simulink model "inverted_pendulum"  (R2021a)
settings: Solver=ode15s  StartTime=0.0  StopTime=35  FixedStep=0.1  RelTol=1e-3  EnableMultiTasking=on
settings Model: Creator=glembrez  LastModifiedBy=gabin
settings SolverCC: AlgebraicLoopSolver=TrustRegion  AutoInsertRateTranBlk=on
settings DataIOCC: LimitDataPoints=on
settings OptimizationCC: LifeSpan=inf
settings DebuggingCC: AllowSymbolicDim=off  SFUnexpectedBacktrackingDiag=warning  SFNoUnconditionalDefaultTransitionDiag=warning  SFExecutionAtInitializationDiag=none  ArithmeticOperatorsInVariantConditions=warning
settings SFSimCC: SimUseLocalCustomCode=off  CustomCodeUndefinedFunction=UseInterfaceOnly
settings RTWCC: RTWUseLocalCustomCode=off
settings CodeAppCC: StateflowObjectComments=on
settings GRTTargetCC: TargetLangStandard=C89/C90 (ANSI)
settings ConfigComp: CovMetricSettings=dw  CovSaveCumulativeToWorkspaceVar=on  CovSaveSingleToWorkspaceVar=on  CovExternalEMLEnable=off  CovSFcnEnable=off

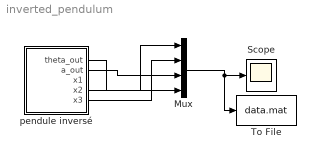
== system inverted_pendulum ==
  Mux : Mux
  Scope : Scope
  To File : ToFile  Filename=data.mat  MatrixName=X  SaveFormat=Timeseries
  pendule inversé : Stateflow chart  TreatAsAtomicUnit=on
  wires:
  Mux/1 -> Scope/1, To File/1
  pendule inversé/1(theta_out) -> Mux/4
  pendule inversé/2(a_out) -> Mux/3
  pendule inversé/4(x2) -> Mux/1
  pendule inversé/5(x3) -> Mux/2

== stateflow chart inverted_pendulum/pendule inversé ==
  settings: updateMethod=CONTINUOUS  sampleTime=0.01
  state Stabilize
    during:
    %computes the derivatives (continuous method)
    x1_dot = x2;
    x2_dot =(m*l*g*sin(x1) - m*l*(-k1*(x1-2*pi*floor((x1+pi)/(2*pi))) - k2*x2)*cos(x1))/J;
    x3_dot = -(-k1*(x1-2*pi*floor((x1+pi)/(2*pi))) -k2*x2)*(l*x2*cos(x1)*m);
    %computes the output (discrete methods)
    theta_out = x1-2*pi*floor((x1+pi)/(2*pi)) ;
    a_out = -k1*(x1-2*pi*floor((x1+pi)/(2*pi))) -k2*x2;
  state Add_energy
    during:
    %computes the derivatives (continuous method)
    x1_dot = x2;
    x2_dot =(m*l*g*sin(x1) -m*l*(-x2*cos(x1))* cos(x1))/J;
    x3_dot = -m*(-x2*cos(x1))*l*x2*cos(x1);
    %computes the output (discrete methods)
    theta_out = x1-2*pi*floor((x1+pi)/(2*pi)) ;
    a_out =-x2*cos(x1);
  state Remove_energy
    during:
    %computes the derivatives (continuous method)
    x1_dot = x2;
    x2_dot =(m*l*g*sin(x1) - m*l*(x2 * cos(x1)) *cos(x1))/J;
    x3_dot = -m*(x2 * cos(x1))*l*x2*cos(x1);
    %computes the output (discrete methods)
    theta_out = x1-2*pi*floor((x1+pi)/(2*pi)) ;
    a_out = x2*cos(x1);
  (default) -> Stabilize : {x1 = -pi;
      | x2 = 0.01;
      | x3 = 0.5*J*x2^2+m*g*l*(cos(x1)-1);
      | e_min = -0;
      | e_max = 5;
      | thetalim = pi/10;}
  Add_energy -> Stabilize [order 2] : [abs(x1-2*pi*floor((x1+pi)/(2*pi)))<thetalim]
  Stabilize -> Remove_energy [order 1] : [abs(x1-2*pi*floor((x1+pi)/(2*pi)))>thetalim &...
      | x3>e_max]
  Stabilize -> Add_energy [order 2] : [abs(x1-2*pi*floor((x1+pi)/(2*pi)))>thetalim &...
      |  x3 < e_min]
  Remove_energy -> Stabilize [order 1] : [abs(x1-2*pi*floor((x1+pi)/(2*pi)))<thetalim]
  Remove_energy -> Add_energy [order 2] : [x3 < e_min]
  Add_energy -> Remove_energy [order 1] : [x3 > e_max]
  data: thetalim local =pi/10; m local =2; g local =9.81; e_min local =-1; e_max local =1; J local =4.5; l local =1.5; theta_out output =-pi; a_out output =0.01; k1 local =-15; k2 local =-3; x1 output =-pi; x2 output =0; x3 output =-1
  data x1 settings: updateMethod=SF_CONTINUOUS_TIME_DATA
  data x2 settings: updateMethod=SF_CONTINUOUS_TIME_DATA
  data x3 settings: updateMethod=SF_CONTINUOUS_TIME_DATA
